simulink model "HIL_Serial_Test"  (R2020a)
settings: Solver=VariableStepAuto  StartTime=0.0  StopTime=10.0  RelTol=1e-3
undefined symbols (not defined in the file): LF, serial
libraries: instrumentlib x3
settings Model: Creator=waldene  LastModifiedBy=waldene

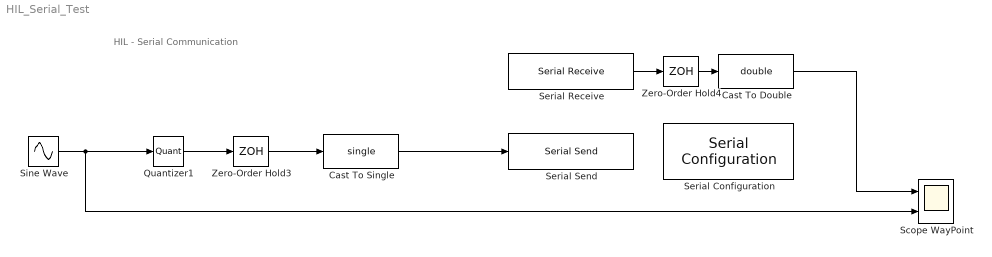
== system HIL_Serial_Test ==
  note: HIL - Serial Communication
  Cast To Double : DataTypeConversion  OutDataTypeStr=double
  Cast To Single : DataTypeConversion  OutDataTypeStr=single
  Quantizer1 : Quantizer  QuantizationInterval=0.01
  Scope WayPoint : Scope  NumInputPorts=2
  Serial Configuration : instrumentlib/Serial Configuration  Priority=-200000  ComPortMenu=<Please select a port...>  ComPort=/dev/ttyUSB0  ObjConstructor=serial('/dev/ttyUSB0');  BaudRate=115200  DataBits=8  Parity=none  StopBits=1  FlowControl=none  Timeout=10  ByteOrder=LittleEndian
  Serial Receive : instrumentlib/Serial Receive  ComPortMenu=<Please select a port...>  ComPort=/dev/ttyUSB0  ObjConstructor=serial('/dev/ttyUSB0');  Header=A  Terminator=LF ('\n')  DataSize="[1  9]"  DataType=single  EnableBlockingMode=on  ActionDataUnavailable=Output last received value  CustomValue=0  SampleTime=0.01
  Serial Send : instrumentlib/Serial Send  ComPortMenu=<Please select a port...>  ComPort=/dev/ttyUSB0  ObjConstructor=serial('/dev/ttyUSB0');  Header=W  Terminator=<none>  EnableBlockingMode=on
  Sine Wave : Sin  SampleTime=0
  Zero-Order Hold3 : ZeroOrderHold  SampleTime=.01
  Zero-Order Hold4 : ZeroOrderHold  SampleTime=.01
  wires:
  Sine Wave/1 -> Scope WayPoint/2, Quantizer1/1
  Serial Receive/1 -> Zero-Order Hold4/1
  Quantizer1/1 -> Zero-Order Hold3/1
  Zero-Order Hold3/1 -> Cast To Single/1
  Cast To Single/1 -> Serial Send/1
  Zero-Order Hold4/1 -> Cast To Double/1
  Cast To Double/1 -> Scope WayPoint/1
